simulink library "dc_motor_lib"  (Simulink 10.2)
settings: Solver=VariableStepAuto  StartTime=0.0  StopTime=10.0  RelTol=1e-3
undefined symbols (not defined in the file): Aobs, Bobs, Cobs, DiscIntNeverNeededParam, Dobs, Kff, L2, Ts
libraries: driveline x6, powerlib x5
settings Model: Creator=raarenst  LastModifiedBy=dirk

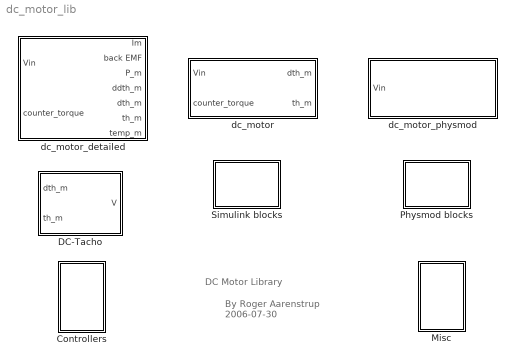
== system dc_motor_lib ==
  note: DC Motor Library
  note: By Roger Aarenstrup
      | 2006-07-30
  Controllers : Subsystem
  DC-Tacho : Subsystem  mask{dth_gain=0.005, th_gain=pi*0.0229, rel_dth_gain=1/486.25}
      mask prompts: dth_gain "Speed Gain (Vs/rad)"; th_gain "Ripple Gain (V/rad)"; rel_dth_gain "Realtive Speed Gain (Vs/rad)"
  Misc : Subsystem
  Physmod blocks : Subsystem
      settings: OpenFcn=sample_physmod_load
      mask Display: disp('Example\nDC Motor\n with load')
  Simulink blocks : Subsystem
      settings: OpenFcn=sample_load
      mask Display: disp('Example\nDC Motor\n with load')
  dc_motor : Subsystem  mask{Rm=2.06, Lm=0.000238, Kb=1/((406*2*pi)/60), Kt=0.0235, Jm=1.07e-6, bm=12e-7}
      mask prompts: Rm "Terminal Resistance (ohms)"; Lm "Terminal inductance (H)"; Kb "Back EMF Constant (Vs/Rad)"; Kt "Torque Constant (Nm/A)"; Jm "Rotor Inertia (Kgm^2)"; bm "Mechanical Damping (Nms/rad)"
  dc_motor_detailed : Subsystem  mask{Rm=2.06, Lm=0.000238, Kb=1/((406*2*pi)/60), Kt=0.0235, Jm=1.07e-6, bm=12e-7, Ktemp=14, ttemp=910, amb_temp=22}
      mask prompts: Rm "Terminal Resistance (ohms)"; Lm "Terminal inductance (H)"; Kb "Back EMF Constant (Vs/Rad)"; Kt "Torque Constant (Nm/A)"; Jm "Rotor Inertia (Kgm^2)"; bm "Mechanical Damping (Nms/rad)"; Ktemp "Thermal Resistance (K/W)"; ttemp "Thermal time constant (s)"; amb_temp "Ambient temperature (C)"
  dc_motor_physmod : Subsystem  mask{Rm=2.06, Lm=0.000238, Kb=1/((406*2*pi)/60), Kt=0.0235, Jm=1.07e-6, bm=12e-7}
      mask prompts: Rm "Terminal Resistance (ohms)"; Lm "Terminal inductance (H)"; Kb "Back EMF Constant (Vs/Rad)"; Kt "Torque Constant (Nm/A)"; Jm "Rotor Inertia (Kgm^2)"; bm "Mechanical Damping (Nms/rad)"

== system dc_motor_lib/Controllers ==
  Discrete PID : Subsystem  mask{K=0.1, b=0.7, Ti=0.01, Td=1e-5, N=4, Tt=0.005, Umax=12, Umin=-12, Ts=Ts}
      mask prompts: K "Proportional Gain (K)"; b "Part of Commanded signal used for P Gain (b)"; Ti "Integral Gain (Ti)"; Td "Derivative Gain (Td)"; N "Derivative Divisor (N)"; Tt "Anti-Windup Gain (Tt)"; Umax "Output Upper Limit (Umax)"; Umin "Output Lower Limit (Umin)"; Ts "Sample Time (Ts)"
      mask Display: disp('DISC\nPID_2')
  Discrete PID1 : Subsystem  mask{K=0.1, b=0.7, Ti=0.01, Td=1e-5, N=4, Ts=Ts}
      mask prompts: K "Proportional Gain (K)"; b "Part of Commanded signal used for P Gain (b)"; Ti "Integral Gain (Ti)"; Td "Derivative Gain (Td)"; N "Derivative Divisor (N)"; Ts "Sample Time (Ts)"
      mask Display: disp('DISC\nPID_1')
  PID approximate derivative1 : Subsystem  mask(PID Controller with approximate derivative){K=0.1, Ti_inv=1/0.03, Td=0.0001, N=3}
      mask prompts: K "Proportional Gain"; Ti_inv "Integral Gain (inverted 1/Ti))"; Td "Derivative Gain"; N "Derivative divisor"
      mask help: This block implements a PID controller with approximate derivative part in the following way: u(s) = K(1 + Ti_inv/s + sTd/(1+sTd/N)) e(s). Note that Ti_inv is the inverse of the commonly u sed Ti parameter. N is the derivative divisor that is used to approximate the derivative part, typical values are 3-20.
      mask Display: disp('CONT\nPID_1')
  PID approximate  output derivative : Subsystem  mask(PID Controller with approximate output derivative){K=0.3, Ti_inv=1/0.03, Td=0.000005, N=3}
      mask prompts: K "Proportional Gain"; Ti_inv "Integral Gain (inverted 1/Ti))"; Td "Derivative Gain"; N "Derivative divisor"
      mask help: This block implements a PID controller with approximate derivative part in the following way: u(s) = K(1e(s) + Ti_inv/s e(s) + sTd/(1+sTd/N) y(s)). Note that Ti_inv is the inverse of the commonly u sed Ti parameter. N is the derivative divisor that is used to approximate the derivative part, typical values are 3-20. Please notw that in this version only the output of the plant is derivied in the derivative part.
      mask Display: disp('CONT\nPID_2')
  State Feedback Controller with Observer and Feed Forward Gain : Subsystem

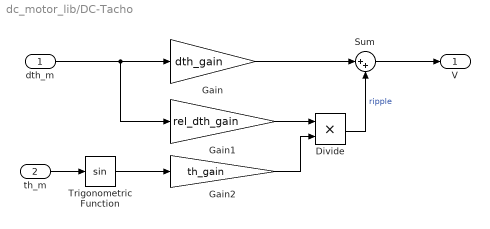
== system dc_motor_lib/DC-Tacho ==
  dth_m : Inport
  th_m : Inport  Port=2
  Divide : Product  Inputs=**
  Gain : Gain  Gain=dth_gain
  Gain1 : Gain  Gain=rel_dth_gain
  Gain2 : Gain  Gain=th_gain
  Sum : Sum  Inputs=|++
  Trigonometric Function : Trigonometry
  V : Outport
  wires:
  Divide/1 -> Sum/2  "ripple"
  Gain1/1 -> Divide/1
  Sum/1 -> V/1
  th_m/1 -> Trigonometric Function/1
  dth_m/1 -> Gain1/1, Gain/1
  Gain2/1 -> Divide/2
  Trigonometric Function/1 -> Gain2/1
  Gain/1 -> Sum/1

== system dc_motor_lib/Misc ==
  10bit : Subsystem
      mask Display: disp('A/D')
  Sample trajectory-generator : Subsystem  mask{aMax=1, tMove=2}
      mask prompts: aMax "Max acceleration [m/s^2]"; tMove "Total movement time [s]"

== system dc_motor_lib/Physmod blocks ==
  Gain : Gain

== system dc_motor_lib/Simulink blocks ==
  Gain : Gain

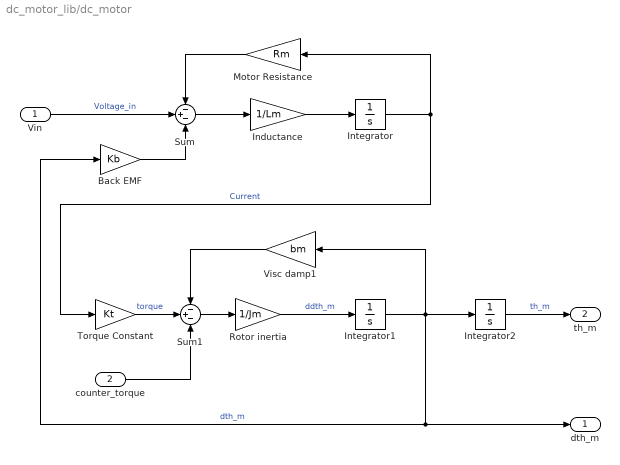
== system dc_motor_lib/dc_motor ==
  Vin : Inport
  counter_torque : Inport  Port=2
  Back EMF : Gain  Gain=Kb
  Inductance : Gain  Gain=1/Lm
  Integrator : Integrator
  Integrator1 : Integrator
  Integrator2 : Integrator
  Motor Resistance : Gain  Gain=Rm
  Rotor inertia : Gain  Gain=1/Jm
  Sum : Sum  Inputs=-+-
  Sum1 : Sum  Inputs=-+-
  Torque Constant : Gain  Gain=Kt
  Visc damp1 : Gain  Gain=bm
  dth_m : Outport
  th_m : Outport  Port=2
  wires:
  Back EMF/1 -> Sum/3
  Motor Resistance/1 -> Sum/1
  Sum/1 -> Inductance/1
  Inductance/1 -> Integrator/1
  Integrator/1 -> Torque Constant/1, Motor Resistance/1  "Current"
  Integrator1/1 -> Visc damp1/1, Integrator2/1, Back EMF/1, dth_m/1  "dth_m"
  Torque Constant/1 -> Sum1/2  "torque"
  Sum1/1 -> Rotor inertia/1
  Rotor inertia/1 -> Integrator1/1  "ddth_m"
  Vin/1 -> Sum/2  "Voltage_in"
  Integrator2/1 -> th_m/1  "th_m"
  Visc damp1/1 -> Sum1/1
  counter_torque/1 -> Sum1/3

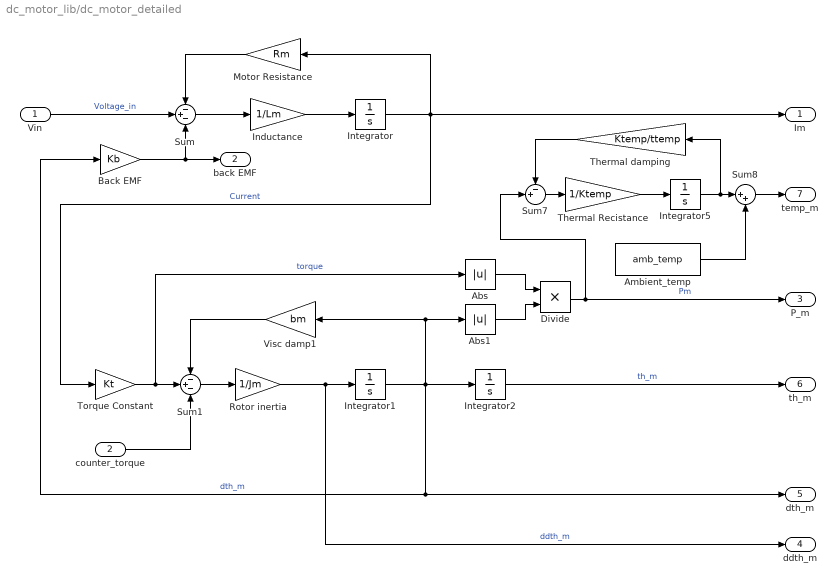
== system dc_motor_lib/dc_motor_detailed ==
  Vin : Inport
  counter_torque : Inport  Port=2
  Abs : Abs
  Abs1 : Abs
  Ambient_temp : Constant  Value=amb_temp  SampleTime=0
  Back EMF : Gain  Gain=Kb
  Divide : Product  Inputs=**
  Inductance : Gain  Gain=1/Lm
  Integrator{,1..2,5} (4 alike) : Integrator
  Motor Resistance : Gain  Gain=Rm
  Rotor inertia : Gain  Gain=1/Jm
  Sum : Sum  Inputs=-+-
  Sum1 : Sum  Inputs=-+-
  Sum7 : Sum  Inputs=-+|
  Sum8 : Sum  Inputs=|++
  Thermal Recistance : Gain  Gain=1/Ktemp
  Thermal damping : Gain  Gain=Ktemp/ttemp
  Torque Constant : Gain  Gain=Kt
  Visc damp1 : Gain  Gain=bm
  Im : Outport
  back EMF : Outport  Port=2
  P_m : Outport  Port=3
  ddth_m : Outport  Port=4
  dth_m : Outport  Port=5
  th_m : Outport  Port=6
  temp_m : Outport  Port=7
  wires:
  counter_torque/1 -> Sum1/3
  Visc damp1/1 -> Sum1/1
  Divide/1 -> Sum7/2, P_m/1  "Pm"
  Sum8/1 -> temp_m/1
  Integrator2/1 -> th_m/1  "th_m"
  Vin/1 -> Sum/2  "Voltage_in"
  Abs1/1 -> Divide/2
  Abs/1 -> Divide/1
  Ambient_temp/1 -> Sum8/2
  Thermal damping/1 -> Sum7/1
  Sum7/1 -> Thermal Recistance/1
  Thermal Recistance/1 -> Integrator5/1
  Integrator5/1 -> Thermal damping/1, Sum8/1
  Rotor inertia/1 -> ddth_m/1, Integrator1/1  "ddth_m"
  Sum1/1 -> Rotor inertia/1
  Torque Constant/1 -> Sum1/2, Abs/1  "torque"
  Integrator1/1 -> dth_m/1, Back EMF/1, Abs1/1, Visc damp1/1, Integrator2/1  "dth_m"
  Integrator/1 -> Im/1, Motor Resistance/1, Torque Constant/1  "Current"
  Inductance/1 -> Integrator/1
  Sum/1 -> Inductance/1
  Motor Resistance/1 -> Sum/1
  Back EMF/1 -> Sum/3, back EMF/1

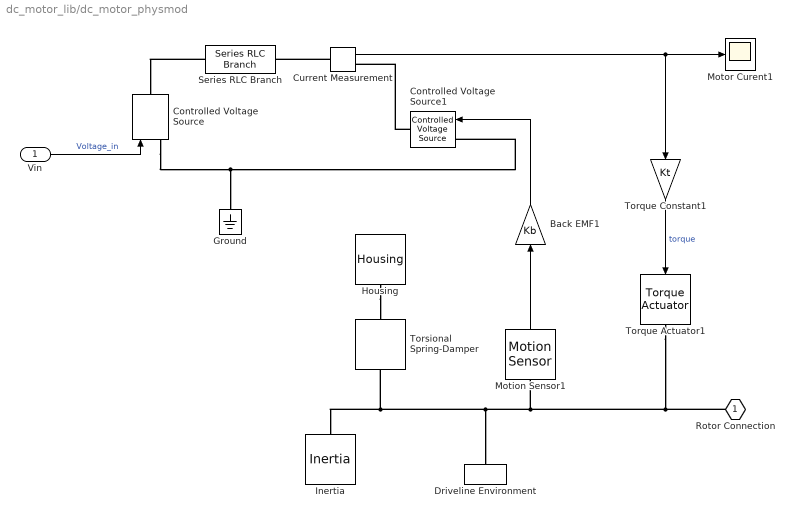
== system dc_motor_lib/dc_motor_physmod ==
  Vin : Inport
  Back EMF1 : Gain  Gain=Kb
  Controlled Voltage Source : powerlib/Electrical Sources/Controlled Voltage Source  SystemSampleTime=-1  Initialize=on  Source_Type=AC  Amplitude=0  Phase=0  Frequency=0  Measurements=None
  Controlled Voltage Source1 : powerlib/Electrical Sources/Controlled Voltage Source  SystemSampleTime=-1  Initialize=off  Source_Type=DC  Amplitude=0  Phase=0  Frequency=0  Measurements=None
  Current Measurement : powerlib/Measurements/Current Measurement  SystemSampleTime=-1  PhasorSimulation=off  OutputType=Complex  PSBequivalent=0
  Driveline Environment : driveline/Solver & Inertias/Driveline Environment  SystemSampleTime=-1  PortType=p1  BlockClass=Solver  PhysicalDomain=driveline_domain  SimulationMode=Dynamics  ModeIteration=on  DefaultUseAutoClutchVelocityTolerance=on  DefaultClutchVelocityTolerance=1e-3
      settings: SourceProductBaseCode=LD
  Ground : powerlib/Elements/Ground  PhysicalDomain=powersysdomain  SubClassName=unknown  LeftPortType=p1  RightPortType=p1  LConnTagsString=a
  Housing : driveline/Solver & Inertias/Housing  SystemSampleTime=-1
      settings: SourceProductBaseCode=LD
  Inertia : driveline/Solver & Inertias/Inertia  SystemSampleTime=-1  PortType=p1  BlockClass=Inertia  PhysicalDomain=driveline_domain  I=Jm  Ip=[]  Iv=[]  ShowLeft=off  ShowRight=on
      settings: SourceProductBaseCode=LD
  Motion Sensor1 : driveline/Sensors & Actuators/Motion Sensor  SystemSampleTime=-1  Angle=off  x0=0  Velocity=on  Acceleration=off
      settings: SourceProductBaseCode=LD
  Motor Curent1 : Scope
  Series RLC Branch : powerlib/Elements/Series RLC Branch  PhysicalDomain=powersysdomain  SubClassName=unknown  LeftPortType=p1  RightPortType=p1  LConnTagsString=__new0  RConnTagsString=__new0  BranchType=RL  Resistance=Rm  Inductance=Lm  SetiL0=off  InitialCurrent=0  Capacitance=1.0  Setx0=off  InitialVoltage=0  Measurements=None
  Torque Actuator1 : driveline/Sensors & Actuators/Torque Actuator  SystemSampleTime=-1
      settings: SourceProductBaseCode=LD
  Torque Constant1 : Gain  Gain=Kt
  Torsional  Spring-Damper : driveline/Dynamic Elements/Torsional  Spring-Damper  SystemSampleTime=-1  k=0  c=bm  x0=0  Backlash=0
      settings: SourceProductBaseCode=LD
  Rotor Connection : PMIOPort  Side=Right
  wires:
  Torque Constant1/1 -> Torque Actuator1/1  "torque"
  Motion Sensor1/1 -> Back EMF1/1
  Back EMF1/1 -> Controlled Voltage Source1/1
  Current Measurement/1 -> Torque Constant1/1, Motor Curent1/1
  Vin/1 -> Controlled Voltage Source/1  "Voltage_in"
  connections:
  Housing/RConn1 -- Torsional  Spring-Damper/RConn1
  Controlled Voltage Source1/RConn1 -- Current Measurement/RConn1
  Current Measurement/LConn1 -- Series RLC Branch/RConn1
  Controlled Voltage Source1/LConn1 -- Ground/LConn1 -- Controlled Voltage Source/LConn1
  Series RLC Branch/LConn1 -- Controlled Voltage Source/RConn1
  Motion Sensor1/LConn1 -- Torque Actuator1/RConn1 -- Rotor Connection/RConn1 -- Inertia/RConn1 -- Torsional  Spring-Damper/LConn1 -- Driveline Environment/LConn1

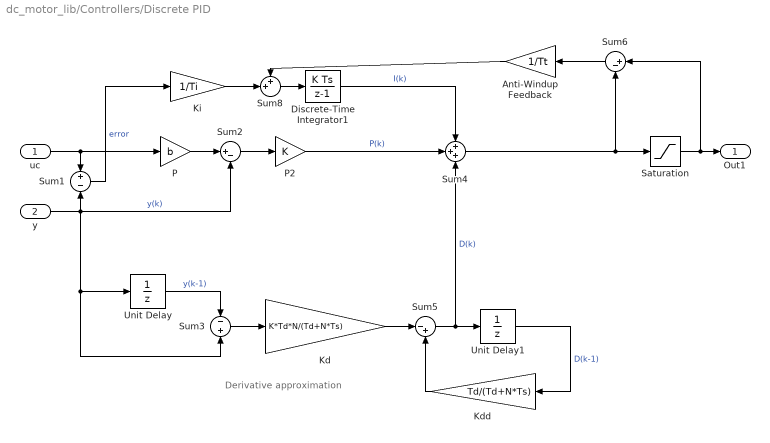
== system dc_motor_lib/Controllers/Discrete PID ==
  note: Derivative approximation
  uc : Inport
  y : Inport  Port=2
  Anti-Windup Feedback : Gain  Gain=1/Tt  SampleTime=Ts
  Discrete-Time Integrator1 : DiscreteIntegrator  gainval=K  SampleTime=Ts  ICPrevOutput=DiscIntNeverNeededParam  ICPrevScaledInput=DiscIntNeverNeededParam
  Kd : Gain  Gain=K*Td*N/(Td+N*Ts)  SampleTime=Ts
  Kdd : Gain  Gain=Td/(Td+N*Ts)  SampleTime=Ts
  Ki : Gain  Gain=1/Ti  SampleTime=Ts
  P : Gain  Gain=b  SampleTime=Ts
  P2 : Gain  Gain=K  SampleTime=Ts
  Saturation : Saturate  UpperLimit=Umax  LowerLimit=Umin  SampleTime=Ts
  Sum1 : Sum  Inputs=+-
  Sum2 : Sum  Inputs=|+-
  Sum3 : Sum  Inputs=-+
  Sum4 : Sum  Inputs=+++
  Sum5 : Sum  Inputs=|-+
  Sum6 : Sum  Inputs=|+-
  Sum8 : Sum  Inputs=++|
  Unit Delay : UnitDelay  SampleTime=Ts
  Unit Delay1 : UnitDelay  SampleTime=Ts
  Out1 : Outport
  wires:
  Kdd/1 -> Sum5/2
  Kd/1 -> Sum5/1
  Unit Delay1/1 -> Kdd/1  "D(k-1)"
  Sum5/1 -> Sum4/3, Unit Delay1/1  "D(k)"
  Sum3/1 -> Kd/1
  Unit Delay/1 -> Sum3/1  "y(k-1)"
  Sum1/1 -> Ki/1  "error"
  Sum2/1 -> P2/1
  y/1 -> Sum3/2, Unit Delay/1, Sum1/2, Sum2/2  "y(k)"
  P/1 -> Sum2/1
  uc/1 -> P/1, Sum1/1
  P2/1 -> Sum4/2  "P(k)"
  Sum4/1 -> Saturation/1, Sum6/2
  Saturation/1 -> Out1/1, Sum6/1
  Discrete-Time Integrator1/1 -> Sum4/1  "I(k)"
  Sum6/1 -> Anti-Windup Feedback/1
  Anti-Windup Feedback/1 -> Sum8/1
  Ki/1 -> Sum8/2
  Sum8/1 -> Discrete-Time Integrator1/1

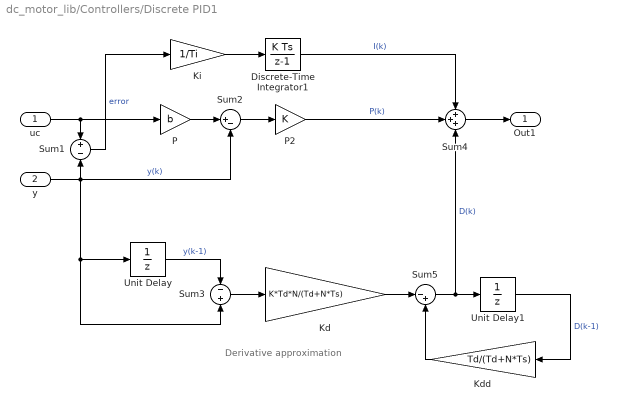
== system dc_motor_lib/Controllers/Discrete PID1 ==
  note: Derivative approximation
  uc : Inport
  y : Inport  Port=2
  Discrete-Time Integrator1 : DiscreteIntegrator  gainval=K  SampleTime=Ts  ICPrevOutput=DiscIntNeverNeededParam  ICPrevScaledInput=DiscIntNeverNeededParam
  Kd : Gain  Gain=K*Td*N/(Td+N*Ts)
  Kdd : Gain  Gain=Td/(Td+N*Ts)
  Ki : Gain  Gain=1/Ti
  P : Gain  Gain=b
  P2 : Gain  Gain=K
  Sum1 : Sum  Inputs=+-
  Sum2 : Sum  Inputs=|+-
  Sum3 : Sum  Inputs=-+
  Sum4 : Sum  Inputs=+++
  Sum5 : Sum  Inputs=|-+
  Unit Delay : UnitDelay  SampleTime=Ts
  Unit Delay1 : UnitDelay  SampleTime=Ts
  Out1 : Outport
  wires:
  Discrete-Time Integrator1/1 -> Sum4/1  "I(k)"
  P2/1 -> Sum4/2  "P(k)"
  uc/1 -> Sum1/1, P/1
  P/1 -> Sum2/1
  y/1 -> Sum2/2, Sum1/2, Unit Delay/1, Sum3/2  "y(k)"
  Sum2/1 -> P2/1
  Sum1/1 -> Ki/1  "error"
  Ki/1 -> Discrete-Time Integrator1/1
  Unit Delay/1 -> Sum3/1  "y(k-1)"
  Sum3/1 -> Kd/1
  Sum5/1 -> Unit Delay1/1, Sum4/3  "D(k)"
  Unit Delay1/1 -> Kdd/1  "D(k-1)"
  Kd/1 -> Sum5/1
  Kdd/1 -> Sum5/2
  Sum4/1 -> Out1/1

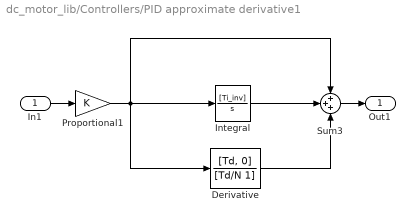
== system dc_motor_lib/Controllers/PID approximate derivative1 ==
  In1 : Inport
  Derivative : TransferFcn  Numerator=[Td, 0]  Denominator=[Td/N 1]
  Integral : TransferFcn  Numerator=[Ti_inv]  Denominator=[1 0]
  Proportional1 : Gain  Gain=K  SaturateOnIntegerOverflow=on  OutDataTypeStr=Inherit: Same as input  ParamDataTypeStr=Inherit: Same as input
  Sum3 : Sum  Inputs=+++
  Out1 : Outport
  wires:
  Proportional1/1 -> Sum3/1, Integral/1, Derivative/1
  Derivative/1 -> Sum3/3
  Integral/1 -> Sum3/2
  In1/1 -> Proportional1/1
  Sum3/1 -> Out1/1

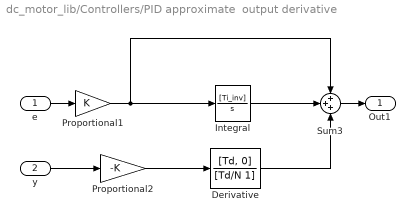
== system dc_motor_lib/Controllers/PID approximate  output derivative ==
  e : Inport
  y : Inport  Port=2
  Derivative : TransferFcn  Numerator=[Td, 0]  Denominator=[Td/N 1]
  Integral : TransferFcn  Numerator=[Ti_inv]  Denominator=[1 0]
  Proportional1 : Gain  Gain=K  SaturateOnIntegerOverflow=on  OutDataTypeStr=Inherit: Same as input  ParamDataTypeStr=Inherit: Same as input
  Proportional2 : Gain  Gain=-K  SaturateOnIntegerOverflow=on  OutDataTypeStr=Inherit: Same as input  ParamDataTypeStr=Inherit: Same as input
  Sum3 : Sum  Inputs=+++
  Out1 : Outport
  wires:
  y/1 -> Proportional2/1
  Proportional2/1 -> Derivative/1
  Proportional1/1 -> Sum3/1, Integral/1
  Derivative/1 -> Sum3/3
  Integral/1 -> Sum3/2
  e/1 -> Proportional1/1
  Sum3/1 -> Out1/1

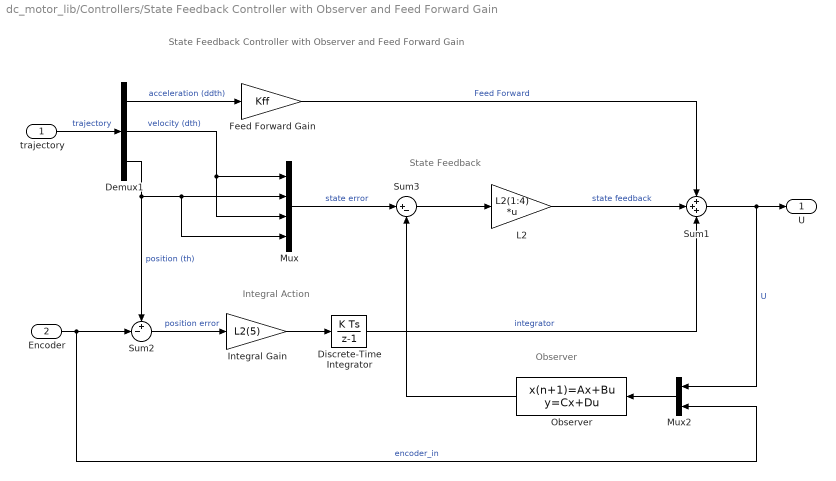
== system dc_motor_lib/Controllers/State Feedback Controller with Observer and Feed Forward Gain ==
  note: Integral Action
  note: State Feedback
  note: Observer
  note: State Feedback Controller with Observer and Feed Forward Gain
  trajectory : Inport
  Encoder : Inport  Port=2
  Demux1 : Demux  Outputs=3
  Discrete-Time Integrator : DiscreteIntegrator  gainval=1  SampleTime=Ts  ICPrevOutput=DiscIntNeverNeededParam  ICPrevScaledInput=DiscIntNeverNeededParam
  Feed Forward Gain : Gain  Gain=Kff  SampleTime=Ts
  Integral Gain : Gain  Gain=L2(5)  SampleTime=Ts
  L2 : Gain  Gain=L2(1:4)  Multiplication=Matrix(K*u) (u vector)  SampleTime=Ts
  Mux : Mux
  Mux2 : Mux  Inputs=2
  Observer : DiscreteStateSpace  A=Aobs  B=Bobs  C=Cobs  D=Dobs  SampleTime=Ts
  Sum1 : Sum  Inputs=+++
  Sum2 : Sum  Inputs=+-|
  Sum3 : Sum  Inputs=|+-
  U : Outport
  wires:
  Observer/1 -> Sum3/2
  Mux2/1 -> Observer/1
  L2/1 -> Sum1/2  "state feedback"
  Demux1/2 -> Mux/3, Mux/1  "velocity (dth)"
  Discrete-Time Integrator/1 -> Sum1/3  "integrator"
  Encoder/1 -> Mux2/2, Sum2/2  "encoder_in"
  Sum1/1 -> Mux2/1, U/1  "U"
  trajectory/1 -> Demux1/1  "trajectory"
  Sum3/1 -> L2/1
  Feed Forward Gain/1 -> Sum1/1  "Feed Forward"
  Mux/1 -> Sum3/1  "state error"
  Demux1/3 -> Mux/4, Mux/2, Sum2/1  "position (th)"
  Demux1/1 -> Feed Forward Gain/1  "acceleration (ddth)"
  Integral Gain/1 -> Discrete-Time Integrator/1
  Sum2/1 -> Integral Gain/1  "position error"

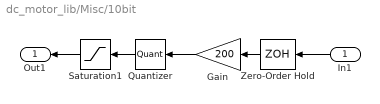
== system dc_motor_lib/Misc/10bit ==
  In1 : Inport
  Gain : Gain  Gain=200
  Quantizer : Quantizer  QuantizationInterval=1  SampleTime=Ts
  Saturation1 : Saturate  UpperLimit=512  LowerLimit=-512  SampleTime=Ts
  Zero-Order Hold : ZeroOrderHold  SampleTime=Ts
  Out1 : Outport
  wires:
  Zero-Order Hold/1 -> Gain/1
  Quantizer/1 -> Saturation1/1
  In1/1 -> Zero-Order Hold/1
  Saturation1/1 -> Out1/1
  Gain/1 -> Quantizer/1

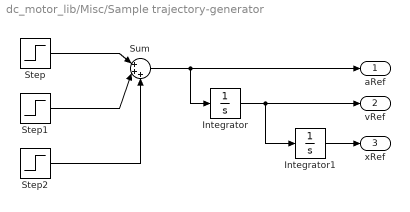
== system dc_motor_lib/Misc/Sample trajectory-generator ==
  Integrator : Integrator
  Integrator1 : Integrator
  Step : Step  Time=0  After=aMax  SampleTime=0
  Step1 : Step  Time=tMove/2  After=-2*aMax  SampleTime=0
  Step2 : Step  Time=2*tMove/2  After=aMax  SampleTime=0
  Sum : Sum  Inputs=|+++  InputSameDT=on  SaturateOnIntegerOverflow=on  OutDataTypeStr=Inherit: Same as first input
  aRef : Outport
  vRef : Outport  Port=2
  xRef : Outport  Port=3
  wires:
  Step/1 -> Sum/1
  Step1/1 -> Sum/2
  Step2/1 -> Sum/3
  Sum/1 -> aRef/1, Integrator/1
  Integrator1/1 -> xRef/1
  Integrator/1 -> vRef/1, Integrator1/1
